simulink library "INT_EBrk_VD"  (R2016b)
settings: Solver=VariableStepAuto  StartTime=0.0  StopTime=10.0  RelTol=1e-3
settings Model: Creator=Administrator  LastModifiedBy=Administrator

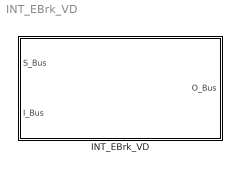
== system INT_EBrk_VD ==
  INT_EBrk_VD : Subsystem

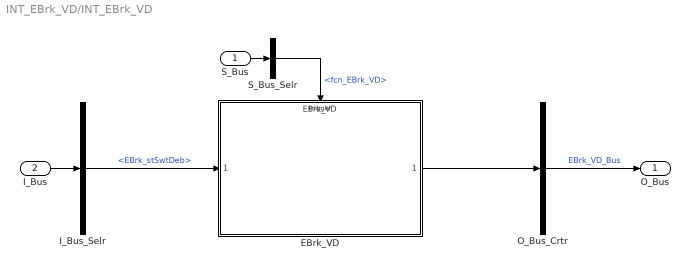
== system INT_EBrk_VD/INT_EBrk_VD ==
  S_Bus : Inport
  I_Bus : Inport  Port=2
  EBrk_VD : ModelReference  ModelNameDialog=EBrk_VD  SimulationMode=Normal  ModelReferenceVersion=1.2  TriggerPortName=function  TriggerPortTriggerType=function-call  TriggerPortStatesWhenEnabling=held
  I_Bus_Selr : BusSelector  OutputSignals=EBrk_stSwtDeb
  O_Bus_Crtr : BusCreator  Inputs=1
  S_Bus_Selr : BusSelector  OutputSignals=fcn_EBrk_VD
  O_Bus : Outport
  wires:
  S_Bus_Selr/1 -> EBrk_VD/Trigger  "<fcn_EBrk_VD>"
  S_Bus/1 -> S_Bus_Selr/1
  I_Bus/1 -> I_Bus_Selr/1
  I_Bus_Selr/1 -> EBrk_VD/1  "<EBrk_stSwtDeb>"
  O_Bus_Crtr/1 -> O_Bus/1  "EBrk_VD_Bus"
  EBrk_VD/1 -> O_Bus_Crtr/1
